simulink model "rw_model"  (R2019b)
settings: Solver=VariableStepAuto  StartTime=0.0  StopTime=600  RelTol=1e-3
values from neighbouring files (symbols this model uses):
  c = 0.0001    [rw_script.m]
  I = 10    [rw_script.m]    (also in thrusters_script.m = 1)
  J = 1    [rw_script.m]
  Kd = 0.1    [rw_script.m]    (also in thrusters_script.m = 2)
  Ki = 0    [rw_script.m]
  Kp = 1    [rw_script.m]    (also in thrusters_script.m = 0.5)
  N = 25e-3    (= 0.025)    [rw_script.m]
  R = 0.1    [rw_script.m]
settings Model: Creator=asmialek  LastModifiedBy=asmialek
settings DataIOCC: SaveOutput=off  SignalLogging=off  DSMLogging=off  ReturnWorkspaceOutputs=off

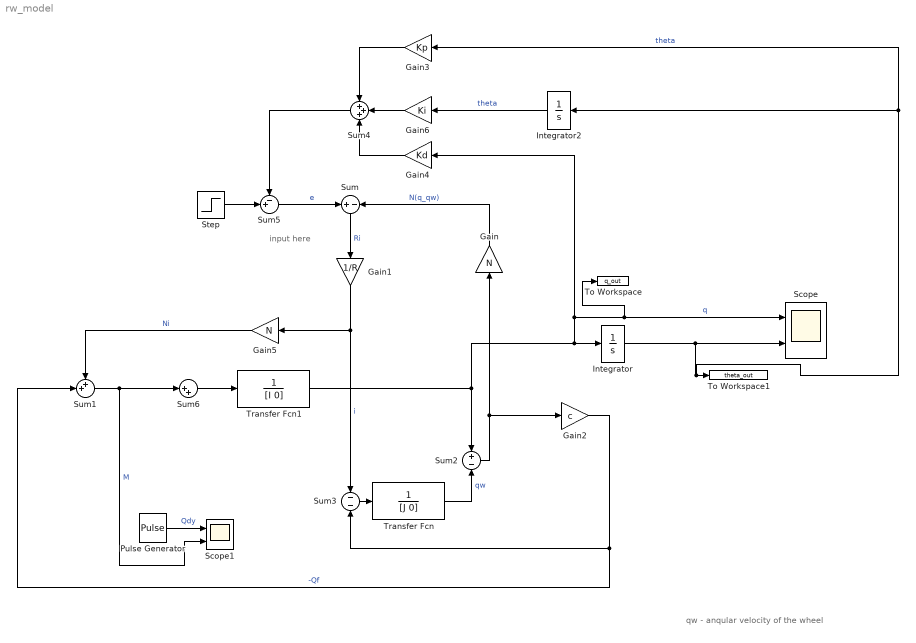
== system rw_model ==
  note: qw - anqular velocity of the wheel
  note: input here
  Gain : Gain  Gain=N
  Gain1 : Gain  Gain=1/R
  Gain2 : Gain  Gain=c
  Gain3 : Gain  Gain=Kp
  Gain4 : Gain  Gain=Kd
  Gain5 : Gain  Gain=N
  Gain6 : Gain  Gain=Ki
  Integrator : Integrator
  Integrator2 : Integrator
  Pulse Generator : DiscretePulseGenerator  PulseType=Time based  Period=200  PulseWidth=0.1
  Scope : Scope  NumInputPorts=2
  Scope1 : Scope  NumInputPorts=2
  Step : Step  Time=20  After=5  SampleTime=0
  Sum : Sum  Inputs=+|-
  Sum1 : Sum  Inputs=++|
  Sum2 : Sum  Inputs=+|-
  Sum3 : Sum  Inputs=-|-
  Sum4 : Sum  Inputs=+++
  Sum5 : Sum  Inputs=-+|
  Sum6 : Sum  Inputs=|++
  To Workspace : ToWorkspace  VariableName=q_out  SampleTime=-1
  To Workspace1 : ToWorkspace  VariableName=theta_out  SampleTime=-1
  Transfer Fcn : TransferFcn  Denominator=[J 0]
  Transfer Fcn1 : TransferFcn  Denominator=[I 0]
  wires:
  Transfer Fcn1/1 -> Integrator/1, Gain4/1, To Workspace/1, Scope/1, Sum2/1  "q"
  Gain/1 -> Sum/2  "N(q_qw)"
  Sum/1 -> Gain1/1  "Ri"
  Gain1/1 -> Sum3/1, Gain5/1  "i"
  Transfer Fcn/1 -> Sum2/2  "qw"
  Sum2/1 -> Gain/1, Gain2/1
  Gain2/1 -> Sum3/2, Sum1/2  "-Qf"
  Gain3/1 -> Sum4/1
  Sum5/1 -> Sum/1  "e"
  Step/1 -> Sum5/2
  Sum4/1 -> Sum5/1
  Gain5/1 -> Sum1/1  "Ni"
  Pulse Generator/1 -> Scope1/1  "Qdy"
  Sum1/1 -> Scope1/2, Sum6/1  "M"
  Gain4/1 -> Sum4/3
  Integrator2/1 -> Gain6/1  "theta"
  Gain6/1 -> Sum4/2
  Integrator/1 -> Gain3/1, Integrator2/1, To Workspace1/1, Scope/2  "theta"
  Sum3/1 -> Transfer Fcn/1
  Sum6/1 -> Transfer Fcn1/1
